simulink model "customsaberdemo"  (Simulink 4.00)
settings: Solver=ode1  StartTime=0.0  StopTime=5  FixedStep=.2  RelTol=1e-3
libraries: simulink3 x1
settings Model: LastModifiedBy=abrooker

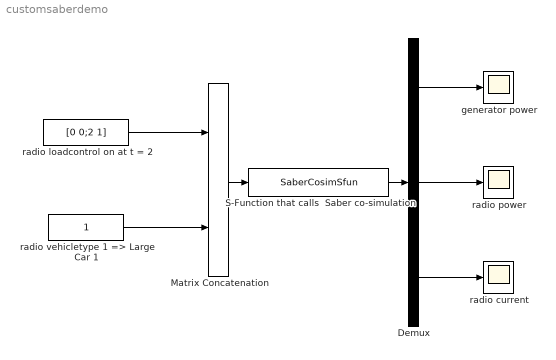
== system customsaberdemo ==
  Demux : Demux  Outputs=3  BusSelectionMode=off
  Matrix Concatenation : simulink3/Signals & Systems/Matrix Concatenation  numInports=2  catMethod=Horizontal
  S-Function that calls  Saber co-simulation : S-Function  FunctionName=SaberCosimSfun  Parameters=strrep(which('advisor'),'advisor.m','tmp\'),.2,'SaberCosimIO_Example'  PortCounts=[]  SFunctionModules=''
  generator power : Scope
      settings: TimeRange=5  YMin=0  YMax=400  SaveToWorkspace=off  SaveName=ScopeData  LimitDataPoints=on  MaxDataPoints=5000
  radio current : Scope
      settings: TimeRange=5  YMin=0  YMax=1.4  SaveToWorkspace=off  SaveName=ScopeData3  LimitDataPoints=on  MaxDataPoints=5000
  radio loadcontrol on at t = 2 : FromWorkspace  VariableName=[0 0;2 1]  SampleTime=0  Interpolate=off  OutputAfterFinalValue=HoldingFinalValue
  radio power : Scope
      settings: TimeRange=5  YMin=0  YMax=20  SaveToWorkspace=off  SaveName=ScopeData2  LimitDataPoints=on  MaxDataPoints=5000
  radio vehicletype 1 => Large Car 1 : Constant  Value=1
  wires:
  radio loadcontrol on at t = 2/1 -> Matrix Concatenation/1
  Matrix Concatenation/1 -> S-Function that calls  Saber co-simulation/1
  radio vehicletype 1 => Large Car 1/1 -> Matrix Concatenation/2
  S-Function that calls  Saber co-simulation/1 -> Demux/1
  Demux/1 -> generator power/1
  Demux/2 -> radio power/1
  Demux/3 -> radio current/1
